simulink model "RLC_ex10"  (R2021b)
settings: Solver=VariableStepAuto  StartTime=0.0  StopTime=10.0  RelTol=1e-3
values from neighbouring files (symbols this model uses):
  D = [ 1,2,4]    [ex10.m]    (also in ex22.m = 0.4; ex23.m = 0.1; ex34.m = [C(2) C(4);d1 0])
  K = 1    [ex10.m]    (also in ex22.m)
  M = 1    [ex10.m]    (also in ex22.m = 5)
settings Model: Creator=rafam  LastModifiedBy=rafam

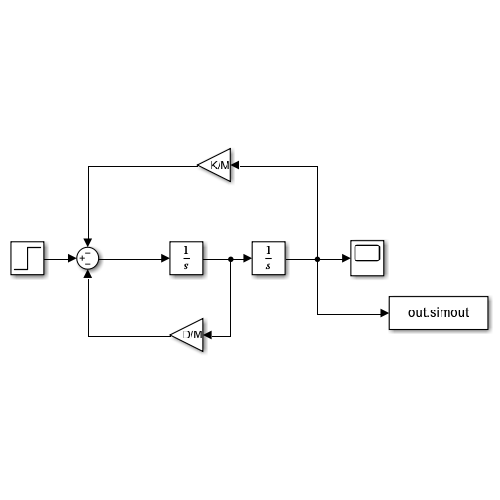
[thumbnail: Simulink's stored preview of the top-level diagram]
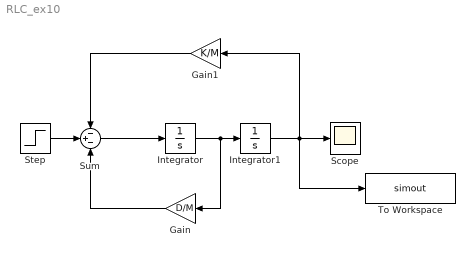
== system RLC_ex10 ==
  Gain : Gain  Gain=D/M
  Gain1 : Gain  Gain=K/M
  Integrator : Integrator
  Integrator1 : Integrator
  Scope : Scope
  Step : Step  Time=0  SampleTime=0
  Sum : Sum  Inputs=-+-
  To Workspace : ToWorkspace  VariableName=simout  SaveFormat=Timeseries  SampleTime=-1
  wires:
  Integrator/1 -> Gain/1, Integrator1/1
  Sum/1 -> Integrator/1
  Gain1/1 -> Sum/1
  Gain/1 -> Sum/3
  Step/1 -> Sum/2
  Integrator1/1 -> To Workspace/1, Gain1/1, Scope/1
